simulink model "FKtest4"  (Simulink 6.6)
settings: Solver=ode4  StartTime=0.0  StopTime=1200  FixedStep=0.05  RelTol=1e-3
undefined symbols (not defined in the file or in its folder): vessel
libraries: simulink x72, marine_gnc x12
(part 3 of 3)

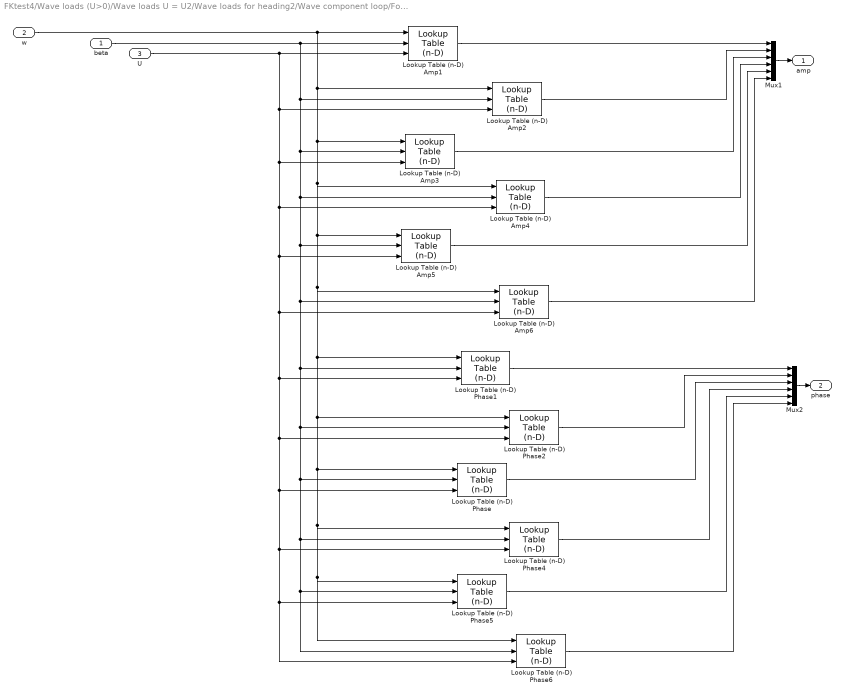
== system FKtest4/Wave loads (U>0)/Wave loads U = U2/Wave loads for heading2/Wave component loop/Force RAO tables ==
  beta : Inport
  w : Inport  Port=2
  U : Inport  Port=3
  Lookup Table (n-D) Amp1 : simulink/Lookup Tables/Lookup Table (n-D)  numDimsPopupSelect=3  bp1=ForceRAO_Freq  bp2=vessel.headings  bp3=RAO_Vel  bp4=[1:3]  bpcell={ [1:3], [1:3] }  explicitNumDims=2  searchMode=Linear Search  cacheBpFlag=on  vectorInputFlag=off  tableData=ForceRAO_Amp{1}  interpMethod=Linear  extrapMethod=None - Clip  rangeErrorMode=Warning
  Lookup Table (n-D) Amp2 : simulink/Lookup Tables/Lookup Table (n-D)  numDimsPopupSelect=3  bp1=ForceRAO_Freq  bp2=vessel.headings  bp3=RAO_Vel  bp4=[1:3]  bpcell={ [1:3], [1:3] }  explicitNumDims=2  searchMode=Linear Search  cacheBpFlag=on  vectorInputFlag=off  tableData=ForceRAO_Amp{2}  interpMethod=Linear  extrapMethod=None - Clip  rangeErrorMode=Warning
  Lookup Table (n-D) Amp3 : simulink/Lookup Tables/Lookup Table (n-D)  numDimsPopupSelect=3  bp1=ForceRAO_Freq  bp2=vessel.headings  bp3=RAO_Vel  bp4=[1:3]  bpcell={ [1:3], [1:3] }  explicitNumDims=2  searchMode=Linear Search  cacheBpFlag=on  vectorInputFlag=off  tableData=ForceRAO_Amp{3}  interpMethod=Linear  extrapMethod=None - Clip  rangeErrorMode=Warning
  Lookup Table (n-D) Amp4 : simulink/Lookup Tables/Lookup Table (n-D)  numDimsPopupSelect=3  bp1=ForceRAO_Freq  bp2=vessel.headings  bp3=RAO_Vel  bp4=[1:3]  bpcell={ [1:3], [1:3] }  explicitNumDims=2  searchMode=Linear Search  cacheBpFlag=on  vectorInputFlag=off  tableData=ForceRAO_Amp{4}  interpMethod=Linear  extrapMethod=None - Clip  rangeErrorMode=Warning
  Lookup Table (n-D) Amp5 : simulink/Lookup Tables/Lookup Table (n-D)  numDimsPopupSelect=3  bp1=ForceRAO_Freq  bp2=vessel.headings  bp3=RAO_Vel  bp4=[1:3]  bpcell={ [1:3], [1:3] }  explicitNumDims=2  searchMode=Linear Search  cacheBpFlag=on  vectorInputFlag=off  tableData=ForceRAO_Amp{5}  interpMethod=Linear  extrapMethod=None - Clip  rangeErrorMode=Warning
  Lookup Table (n-D) Amp6 : simulink/Lookup Tables/Lookup Table (n-D)  numDimsPopupSelect=3  bp1=ForceRAO_Freq  bp2=vessel.headings  bp3=RAO_Vel  bp4=[1:3]  bpcell={ [1:3], [1:3] }  explicitNumDims=2  searchMode=Linear Search  cacheBpFlag=on  vectorInputFlag=off  tableData=ForceRAO_Amp{6}  interpMethod=Linear  extrapMethod=None - Clip  rangeErrorMode=Warning
  Lookup Table (n-D) Phase : simulink/Lookup Tables/Lookup Table (n-D)  numDimsPopupSelect=3  bp1=ForceRAO_Freq  bp2=vessel.headings  bp3=RAO_Vel  bp4=[1:3]  bpcell={ [1:3], [1:3] }  explicitNumDims=2  searchMode=Linear Search  cacheBpFlag=on  vectorInputFlag=off  tableData=ForceRAO_Phase{3}  interpMethod=Linear  extrapMethod=None - Clip  rangeErrorMode=Warning
  Lookup Table (n-D) Phase1 : simulink/Lookup Tables/Lookup Table (n-D)  numDimsPopupSelect=3  bp1=ForceRAO_Freq  bp2=vessel.headings  bp3=RAO_Vel  bp4=[1:3]  bpcell={ [1:3], [1:3] }  explicitNumDims=2  searchMode=Linear Search  cacheBpFlag=on  vectorInputFlag=off  tableData=ForceRAO_Phase{1}  interpMethod=Linear  extrapMethod=None - Clip  rangeErrorMode=Warning
  Lookup Table (n-D) Phase2 : simulink/Lookup Tables/Lookup Table (n-D)  numDimsPopupSelect=3  bp1=ForceRAO_Freq  bp2=vessel.headings  bp3=RAO_Vel  bp4=[1:3]  bpcell={ [1:3], [1:3] }  explicitNumDims=2  searchMode=Linear Search  cacheBpFlag=on  vectorInputFlag=off  tableData=ForceRAO_Phase{2}  interpMethod=Linear  extrapMethod=None - Clip  rangeErrorMode=Warning
  Lookup Table (n-D) Phase4 : simulink/Lookup Tables/Lookup Table (n-D)  numDimsPopupSelect=3  bp1=ForceRAO_Freq  bp2=vessel.headings  bp3=RAO_Vel  bp4=[1:3]  bpcell={ [1:3], [1:3] }  explicitNumDims=2  searchMode=Linear Search  cacheBpFlag=on  vectorInputFlag=off  tableData=ForceRAO_Phase{4}  interpMethod=Linear  extrapMethod=None - Clip  rangeErrorMode=Warning
  Lookup Table (n-D) Phase5 : simulink/Lookup Tables/Lookup Table (n-D)  numDimsPopupSelect=3  bp1=ForceRAO_Freq  bp2=vessel.headings  bp3=RAO_Vel  bp4=[1:3]  bpcell={ [1:3], [1:3] }  explicitNumDims=2  searchMode=Linear Search  cacheBpFlag=on  vectorInputFlag=off  tableData=ForceRAO_Phase{5}  interpMethod=Linear  extrapMethod=None - Clip  rangeErrorMode=Warning
  Lookup Table (n-D) Phase6 : simulink/Lookup Tables/Lookup Table (n-D)  numDimsPopupSelect=3  bp1=ForceRAO_Freq  bp2=vessel.headings  bp3=RAO_Vel  bp4=[1:3]  bpcell={ [1:3], [1:3] }  explicitNumDims=2  searchMode=Linear Search  cacheBpFlag=on  vectorInputFlag=off  tableData=ForceRAO_Phase{6}  interpMethod=Linear  extrapMethod=None - Clip  rangeErrorMode=Warning
  Mux1 : Mux  Inputs=6
  Mux2 : Mux  Inputs=6
  amp : Outport
  phase : Outport  Port=2
  wires:
  w/1 -> Lookup Table (n-D) Amp1/1, Lookup Table (n-D) Amp2/1, Lookup Table (n-D) Amp3/1, Lookup Table (n-D) Amp4/1, Lookup Table (n-D) Amp5/1, Lookup Table (n-D) Amp6/1, Lookup Table (n-D) Phase1/1, Lookup Table (n-D) Phase2/1, Lookup Table (n-D) Phase/1, Lookup Table (n-D) Phase4/1, Lookup Table (n-D) Phase6/1, Lookup Table (n-D) Phase5/1
  Lookup Table (n-D) Phase5/1 -> Mux2/5
  Lookup Table (n-D) Phase/1 -> Mux2/3
  Lookup Table (n-D) Phase1/1 -> Mux2/1
  beta/1 -> Lookup Table (n-D) Amp1/2, Lookup Table (n-D) Amp2/2, Lookup Table (n-D) Amp3/2, Lookup Table (n-D) Amp4/2, Lookup Table (n-D) Amp5/2, Lookup Table (n-D) Amp6/2, Lookup Table (n-D) Phase1/2, Lookup Table (n-D) Phase2/2, Lookup Table (n-D) Phase/2, Lookup Table (n-D) Phase4/2, Lookup Table (n-D) Phase6/2, Lookup Table (n-D) Phase5/2
  Lookup Table (n-D) Phase4/1 -> Mux2/4
  Lookup Table (n-D) Phase2/1 -> Mux2/2
  Lookup Table (n-D) Phase6/1 -> Mux2/6
  Lookup Table (n-D) Amp4/1 -> Mux1/4
  U/1 -> Lookup Table (n-D) Amp1/3, Lookup Table (n-D) Amp2/3, Lookup Table (n-D) Amp3/3, Lookup Table (n-D) Amp4/3, Lookup Table (n-D) Amp5/3, Lookup Table (n-D) Amp6/3, Lookup Table (n-D) Phase1/3, Lookup Table (n-D) Phase2/3, Lookup Table (n-D) Phase/3, Lookup Table (n-D) Phase4/3, Lookup Table (n-D) Phase6/3, Lookup Table (n-D) Phase5/3
  Lookup Table (n-D) Amp1/1 -> Mux1/1
  Lookup Table (n-D) Amp3/1 -> Mux1/3
  Lookup Table (n-D) Amp5/1 -> Mux1/5
  Lookup Table (n-D) Amp2/1 -> Mux1/2
  Lookup Table (n-D) Amp6/1 -> Mux1/6
  Mux2/1 -> phase/1
  Mux1/1 -> amp/1

== system FKtest4/Wave loads (U>0)/Wave loads U = U2/Wave loads for heading2/Wave component loop/WD RAO tables ==
  beta : Inport
  w : Inport  Port=2
  U : Inport  Port=3
  Constant : Constant  Value=0
  Lookup Table (n-D)  Wavedrift 1 : simulink/Lookup Tables/Lookup Table (n-D)  numDimsPopupSelect=3  bp1=WD_Freq  bp2=vessel.headings  bp3=RAO_Vel  bp4=[1:3]  bpcell={ [1:3], [1:3] }  explicitNumDims=2  searchMode=Linear Search  cacheBpFlag=on  vectorInputFlag=off  tableData=WD_Amp{1}  interpMethod=Linear  extrapMethod=None - Clip  rangeErrorMode=Warning
  Lookup Table (n-D)  Wavedrift 2 : simulink/Lookup Tables/Lookup Table (n-D)  numDimsPopupSelect=3  bp1=WD_Freq  bp2=vessel.headings  bp3=RAO_Vel  bp4=[1:3]  bpcell={ [1:3], [1:3] }  explicitNumDims=2  searchMode=Linear Search  cacheBpFlag=on  vectorInputFlag=off  tableData=WD_Amp{2}  interpMethod=Linear  extrapMethod=None - Clip  rangeErrorMode=Warning
  Lookup Table (n-D)  Wavedrift 3 : simulink/Lookup Tables/Lookup Table (n-D)  numDimsPopupSelect=3  bp1=WD_Freq  bp2=vessel.headings  bp3=RAO_Vel  bp4=[1:3]  bpcell={ [1:3], [1:3] }  explicitNumDims=2  searchMode=Linear Search  cacheBpFlag=on  vectorInputFlag=off  tableData=WD_Amp{3}  interpMethod=Linear  extrapMethod=None - Clip  rangeErrorMode=Warning
  Mux1 : Mux  Inputs=6
  amp : Outport
  wires:
  w/1 -> Lookup Table (n-D)  Wavedrift 1/1, Lookup Table (n-D)  Wavedrift 3/1, Lookup Table (n-D)  Wavedrift 2/1
  Constant/1 -> Mux1/5, Mux1/4, Mux1/3
  beta/1 -> Lookup Table (n-D)  Wavedrift 1/2, Lookup Table (n-D)  Wavedrift 3/2, Lookup Table (n-D)  Wavedrift 2/2
  U/1 -> Lookup Table (n-D)  Wavedrift 1/3, Lookup Table (n-D)  Wavedrift 3/3, Lookup Table (n-D)  Wavedrift 2/3
  Lookup Table (n-D)  Wavedrift 1/1 -> Mux1/1
  Lookup Table (n-D)  Wavedrift 2/1 -> Mux1/2
  Lookup Table (n-D)  Wavedrift 3/1 -> Mux1/6
  Mux1/1 -> amp/1

== system FKtest4/Wave loads (U>0)/Wave loads U = U2/Wave loads for heading2/Wave component loop/[-pi pi] to [0 2pi] ==
  note: x
  x [-pi pi] : Inport
  Constant : Constant  Value=2*pi
  Constant1 : Constant  Value=0
  Sign : Signum
  Sum : Sum  Inputs=|++  SaturateOnIntegerOverflow=on
  Switch : Switch
  0<y<2pi : Outport
  wires:
  Constant1/1 -> Switch/1
  Constant/1 -> Switch/3
  Sign/1 -> Switch/2
  Sum/1 -> 0<y<2pi/1
  Switch/1 -> Sum/1
  x [-pi pi]/1 -> Sum/2, Sign/1
